simulink model "QUESTION4_1"  (R2021a)
settings: Solver=VariableStepAuto  StartTime=0.0  StopTime=10.0  RelTol=1e-3
settings Model: Creator=user  LastModifiedBy=user

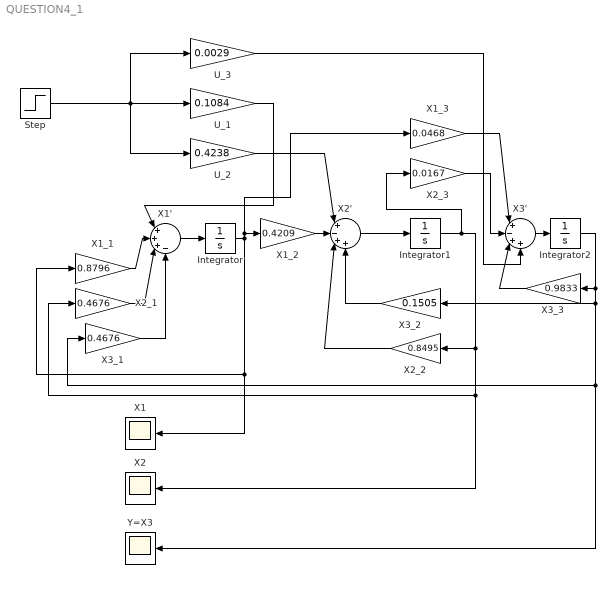
== system QUESTION4_1 ==
  Integrator : Integrator
  Integrator1 : Integrator
  Integrator2 : Integrator
  Step : Step  SampleTime=0
  U_1 : Gain  Gain=0.1084
  U_2 : Gain  Gain=0.4238
  U_3 : Gain  Gain=0.0029
  X1 : Scope
  X1' : Sum  Inputs=|+++-
  X1_1 : Gain  Gain=0.8796
  X1_2 : Gain  Gain=0.4209
  X1_3 : Gain  Gain=0.0468
  X2 : Scope
  X2' : Sum  Inputs=|+-++
  X2_1 : Gain  Gain=0.4676
  X2_2 : Gain  Gain=0.8495
  X2_3 : Gain  Gain=0.0167
  X3' : Sum  Inputs=|+-++
  X3_1 : Gain  Gain=0.4676
  X3_2 : Gain  Gain=0.1505
  X3_3 : Gain  Gain=0.9833
  Y=X3 : Scope
  wires:
  Integrator1/1 -> X2_3/1, X2_2/1, X2_1/1, X2/1
  X3'/1 -> Integrator2/1
  X1'/1 -> Integrator/1
  Integrator2/1 -> X3_3/1, X3_1/1, Y=X3/1, X3_2/1
  X2'/1 -> Integrator1/1
  Step/1 -> U_3/1, U_1/1, U_2/1
  U_2/1 -> X2'/1
  X3_2/1 -> X2'/4
  X2_2/1 -> X2'/3
  X1_2/1 -> X2'/2
  X2_3/1 -> X3'/2
  Integrator/1 -> X1_3/1, X1_2/1, X1/1, X1_1/1
  X1_3/1 -> X3'/1
  U_1/1 -> X1'/1
  X3_1/1 -> X1'/4
  X2_1/1 -> X1'/3
  X1_1/1 -> X1'/2
  X3_3/1 -> X3'/3
  U_3/1 -> X3'/4
